simulink model "Wrist"  (R2020b)
settings: Solver=FixedStepAuto  StartTime=0.0  StopTime=40  RelTol=1e-3
undefined symbols (not defined in the file or in its folder): DiscIntNeverNeededParam
libraries: dspfdesign x2, androidsensorlib x1, simulink x1, vrlib x1
settings Model: SimulationMode=external  Creator=sarar  LastModifiedBy=sarar
settings OptimizationCC: EnhancedBackFolding=on  PassReuseOutputArgsAs=Individual arguments  ZeroExternalMemoryAtStartup=off  ZeroInternalMemoryAtStartup=off  MaxStackSize=64  OptimizeBlockOrder=speed  DifferentSizesBufferReuse=on  OptimizationCustomize=off  EfficientTunableParamExpr=on
settings DebuggingCC: ParameterTunabilityLossMsg=error
settings HardwareCC: ProdBitPerPointer=32  ProdBitPerSizeT=32  ProdBitPerPtrDiffT=32  ProdLargestAtomicInteger=Long  ProdLargestAtomicFloat=Double  ProdWordSize=32  ProdHWDeviceType=ARM Compatible->ARM Cortex
settings SFSimCC: MATLABDynamicMemAlloc=off
settings RTWCC: Description=Embedded Coder  SystemTargetFile=ert.tlc  HardwareBoard=Android Device  TLCOptions="-aInlineSetEventsForThisBaseRateFcn=TLC_FALSE -aSuppressMultiTaskScheduler=TLC_FALSE  -aRateBasedStepFcn=0"  TemplateMakefile=ert_default_tmf  RTWVerbose=off  Toolchain=Android SDK/NDK Tools
settings CodeAppCC: ForceParamTrailComments=on  IgnoreCustomStorageClasses=off  OperatorAnnotations=on  SimulinkDataObjDesc=on  SFDataObjDesc=on  InsertBlockDesc=on

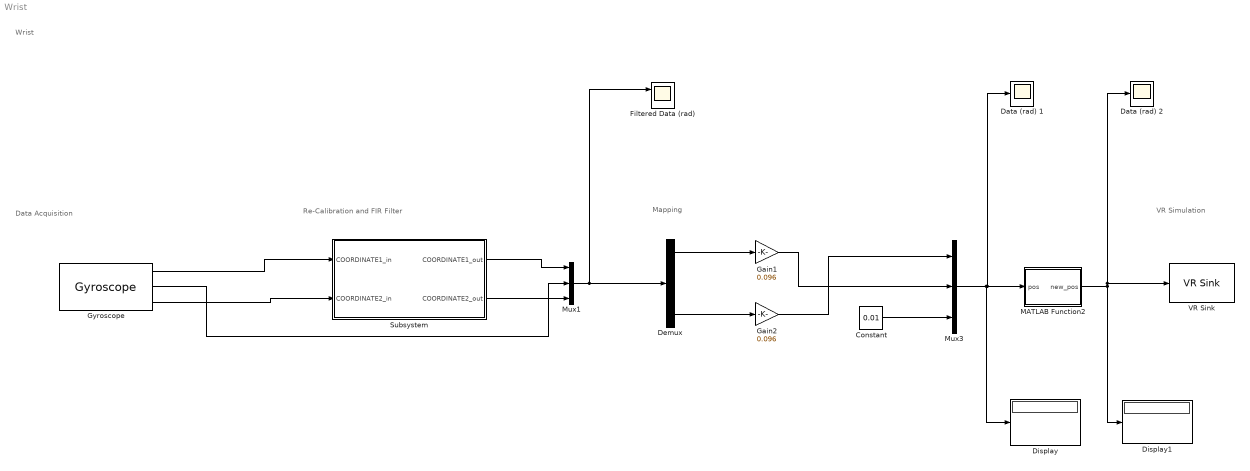
== system Wrist ==
  note: Re-Calibration and FIR Filter
  note: Data Acquisition
  note: Mapping
  note: VR Simulation
  note: Wrist
  Constant : Constant  Value=0.01
  Data (rad) 1 : Scope
  Data (rad) 2 : Scope
  Demux : Demux  Outputs=3
  Display : Display
  Display1 : Display
  Filtered Data (rad) : Scope  NumInputPorts=2
  Gain1 : Gain  Gain=0.096  OutDataTypeStr=Inherit: Inherit via back propagation
  Gain2 : Gain  Gain=0.096  OutDataTypeStr=Inherit: Inherit via back propagation
  Gyroscope : androidsensorlib/Gyroscope  OutputVector=off  SampleTime=0.1  BlockPlatform=Android
      settings: SourceProductBaseCode=ANDROID
  MATLAB Function2 : MATLAB Function  TreatAsAtomicUnit=on
  Mux1 : Mux  Inputs=3
  Mux3 : Mux  Inputs=3
  Subsystem : Subsystem
  VR Sink : vrlib/VR Sink  InstantiateOnLoad=on  SampleTime=0.1  ViewEnable=on  RemoteChange=off  RemoteView=off  FieldsWritten=cursor.translation.3.1.1.double  WorldFileName=8_palline_color.wrl  AutoView=on  VideoDimensions=[]  AllowVariableSize=off
  wires:
  Demux/1 -> Gain1/1
  MATLAB Function2/1(new_pos) -> VR Sink/1, Data (rad) 2/1, Display1/1
  Mux3/1 -> Display/1, MATLAB Function2/1(pos), Data (rad) 1/1
  Mux1/1 -> Demux/1, Filtered Data (rad)/1
  Subsystem/1(COORDINATE1_out) -> Mux1/1
  Gyroscope/1 -> Subsystem/1(COORDINATE1_in)
  Demux/3 -> Gain2/1
  Gain2/1 -> Mux3/1
  Gain1/1 -> Mux3/2
  Constant/1 -> Mux3/3
  Gyroscope/3 -> Subsystem/2(COORDINATE2_in)
  Subsystem/2(COORDINATE2_out) -> Mux1/3
  Gyroscope/2 -> Mux1/2

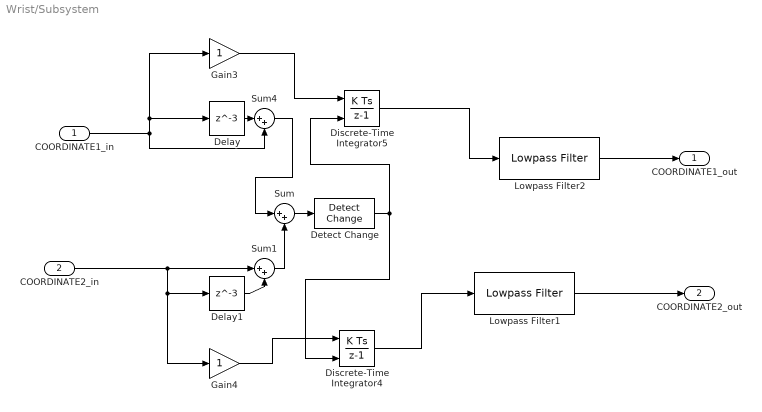
== system Wrist/Subsystem ==
  COORDINATE1_in : Inport
  COORDINATE2_in : Inport  Port=2
  Delay : Delay  DelayLength=3  InitialCondition=0
  Delay1 : Delay  DelayLength=3  InitialCondition=0
  Detect Change : simulink/Logic and Bit Operations/Detect Change  vinit=0  OutDataTypeStr=boolean
  Discrete-Time Integrator4 : DiscreteIntegrator  ExternalReset=either  SampleTime=-1  ICPrevOutput=DiscIntNeverNeededParam  ICPrevScaledInput=DiscIntNeverNeededParam
  Discrete-Time Integrator5 : DiscreteIntegrator  ExternalReset=either  SampleTime=-1  ICPrevOutput=DiscIntNeverNeededParam  ICPrevScaledInput=DiscIntNeverNeededParam
  Gain3 : Gain
  Gain4 : Gain
  Lowpass Filter1 : dspfdesign/Lowpass Filter  FilterType=FIR  DesignForMinimumOrder=on  FilterOrder=5  PassbandFrequency=1  StopbandFrequency=3  PassbandRipple=0.1  StopbandAttenuation=50  InheritSampleRate=off  SampleRate=10  SimulateUsing=Interpreted execution  roundingMode=Floor  coeffsDataTypeStr=fixdt(1,16)
  Lowpass Filter2 : dspfdesign/Lowpass Filter  FilterType=FIR  DesignForMinimumOrder=on  FilterOrder=5  PassbandFrequency=1  StopbandFrequency=3  PassbandRipple=0.1  StopbandAttenuation=50  InheritSampleRate=off  SampleRate=10  SimulateUsing=Interpreted execution  roundingMode=Floor  coeffsDataTypeStr=fixdt(1,16)
  Sum : Sum  Inputs=|++
  Sum1 : Sum  Inputs=|++
  Sum4 : Sum  Inputs=|++
  COORDINATE1_out : Outport
  COORDINATE2_out : Outport  Port=2
  wires:
  Delay/1 -> Sum4/1
  Sum4/1 -> Sum/1
  Delay1/1 -> Sum1/2
  Gain3/1 -> Discrete-Time Integrator5/1
  COORDINATE2_in/1 -> Sum1/1, Gain4/1, Delay1/1
  Sum/1 -> Detect Change/1
  Discrete-Time Integrator4/1 -> Lowpass Filter1/1
  Detect Change/1 -> Discrete-Time Integrator5/2, Discrete-Time Integrator4/2
  Discrete-Time Integrator5/1 -> Lowpass Filter2/1
  Sum1/1 -> Sum/2
  Gain4/1 -> Discrete-Time Integrator4/1
  Lowpass Filter2/1 -> COORDINATE1_out/1
  Lowpass Filter1/1 -> COORDINATE2_out/1
  COORDINATE1_in/1 -> Sum4/2, Delay/1, Gain3/1

== matlab function Wrist/MATLAB Function2 ==
  data: pos input; new_pos output
function new_pos = map(pos)

new_pos = double(pos); 
%define theta 
theta = atan2(pos(2),pos(1)); 


if norm(pos(1)) > norm(0.1*cos(theta))
    new_pos(1) = 0.1 * cos(theta)   
else
    new_pos(1) = pos(1)
end

if norm(pos(2)) > norm(0.1*sin(theta))
    new_pos(2) = 0.1 * sin(theta) 
else
    new_pos(2) = pos(2) 
end 

new_pos(3) = pos(3) 


end
